simulink model "TST_RWSWV2"  (Simulink 10.1)
settings: Solver=FixedStepAuto  StartTime=0.0  StopTime=5.256e+6  FixedStep=1  RelTol=1e-3
libraries: LIB_ROT x3, vrlib x2, dspmathops x2, DYN x1
settings Model: Creator=WilTravis  LastModifiedBy=m_mam
settings DataIOCC: SaveFormat=Dataset
settings OptimizationCC: LifeSpan=auto
settings DebuggingCC: UnderspecifiedInitializationDetection=Simplified  MergeDetectMultiDrivingBlocksExec=error  SFUnexpectedBacktrackingDiag=error  SFNoUnconditionalDefaultTransitionDiag=error  SFExecutionAtInitializationDiag=warning
settings HardwareCC: ProdBitPerLong=64  ProdBitPerPointer=64  ProdBitPerSizeT=64  ProdBitPerPtrDiffT=64  ProdIntDivRoundTo=Zero  ProdEndianess=LittleEndian  ProdWordSize=64  ProdHWDeviceType=AMD->Athlon 64
settings ModelReferenceCC: PropagateSignalLabelsOutOfModel=on
settings CodeAppCC: StateflowObjectComments=off
settings GRTTargetCC: TargetLangStandard=C99 (ISO)  CombineOutputUpdateFcns=on  GRTInterface=off
settings ConfigComp: CovMetricSettings=dwe  CovHtmlReporting=off  CovSaveCumulativeToWorkspaceVar=off  CovSaveSingleToWorkspaceVar=off  CovExternalEMLEnable=on

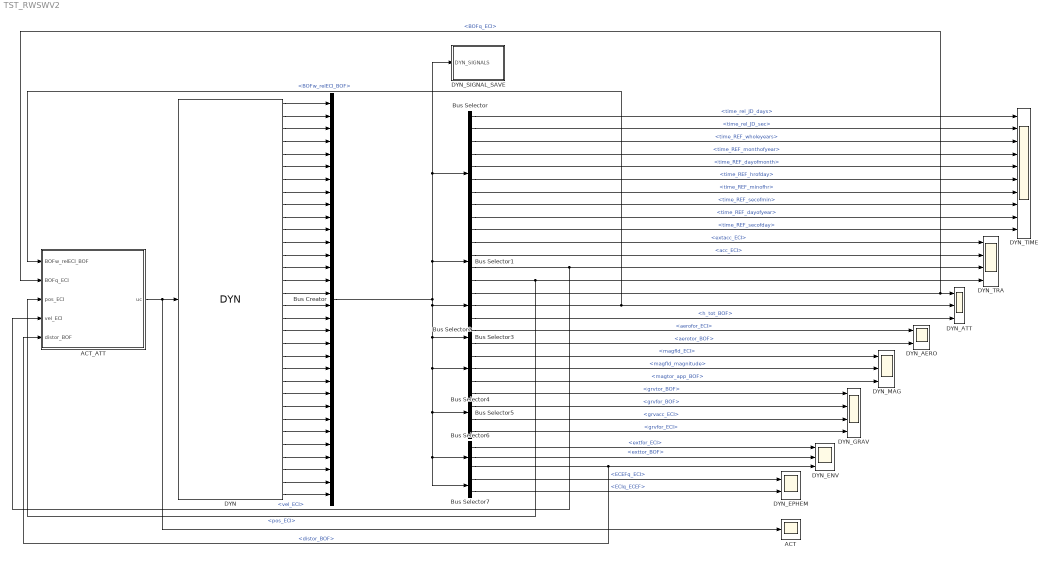
== system TST_RWSWV2 ==
  ACT : Scope
  ACT_ATT : Subsystem
  Bus Creator : BusCreator  Inputs=32
  Bus Selector : BusSelector  OutputSignals=time_rel_JD_days,time_rel_JD_sec,time_REF_wholeyears,time_REF_monthofyear,time_REF_dayofmonth,time_REF_hrofday,time_REF_minofhr,time_REF_secofmin,time_REF_dayofyear,time_REF_secofday
  Bus Selector1 : BusSelector  OutputSignals=extacc_ECI,acc_ECI,vel_ECI,pos_ECI
  Bus Selector2 : BusSelector  OutputSignals=BOFq_ECI,BOFw_relECI_BOF,h_tot_BOF
  Bus Selector3 : BusSelector  OutputSignals=aerofor_ECI,aerotor_BOF
  Bus Selector4 : BusSelector  OutputSignals=magfld_ECI,magfld_magnitude,magtor_app_BOF
  Bus Selector5 : BusSelector  OutputSignals=grvtor_BOF,grvfor_BOF,grvacc_ECI,grvfor_ECI
  Bus Selector6 : BusSelector  OutputSignals=extfor_ECI,exttor_BOF,distor_BOF
  Bus Selector7 : BusSelector  OutputSignals=ECEFq_ECI,ECIq_ECEF
  DYN : DYN/DYN  SystemSampleTime=-1  Latency=0  AutoFrameSizeCalculation=off
  DYN_AERO : Scope  NumInputPorts=2
  DYN_ATT : Scope  NumInputPorts=3
  DYN_ENV : Scope  NumInputPorts=3
  DYN_EPHEM : Scope  NumInputPorts=2
  DYN_GRAV : Scope  NumInputPorts=4
  DYN_MAG : Scope  NumInputPorts=3
  DYN_SIGNAL_SAVE : Subsystem
  DYN_TIME : Scope  NumInputPorts=10
  DYN_TRA : Scope  NumInputPorts=4
  wires:
  Bus Selector4/1 -> DYN_MAG/1  "<magfld_ECI>"
  Bus Selector1/2 -> DYN_TRA/2  "<acc_ECI>"
  Bus Selector/2 -> DYN_TIME/2  "<time_rel_JD_sec>"
  Bus Selector/6 -> DYN_TIME/6  "<time_REF_hrofday>"
  Bus Selector5/1 -> DYN_GRAV/1  "<grvtor_BOF>"
  Bus Selector1/3 -> ACT_ATT/4(vel_ECI), DYN_TRA/3  "<vel_ECI>"
  Bus Selector1/1 -> DYN_TRA/1  "<extacc_ECI>"
  Bus Selector2/1 -> ACT_ATT/2(BOFq_ECI), DYN_ATT/1  "<BOFq_ECI>"
  Bus Selector3/2 -> DYN_AERO/2  "<aerotor_BOF>"
  Bus Selector/3 -> DYN_TIME/3  "<time_REF_wholeyears>"
  Bus Selector5/2 -> DYN_GRAV/2  "<grvfor_BOF>"
  Bus Selector/4 -> DYN_TIME/4  "<time_REF_monthofyear>"
  Bus Selector5/3 -> DYN_GRAV/3  "<grvacc_ECI>"
  Bus Selector3/1 -> DYN_AERO/1  "<aerofor_ECI>"
  Bus Selector/1 -> DYN_TIME/1  "<time_rel_JD_days>"
  Bus Selector/10 -> DYN_TIME/10  "<time_REF_secofday>"
  Bus Selector/7 -> DYN_TIME/7  "<time_REF_minofhr>"
  Bus Selector/8 -> DYN_TIME/8  "<time_REF_secofmin>"
  Bus Selector2/3 -> DYN_ATT/3  "<h_tot_BOF>"
  Bus Selector1/4 -> ACT_ATT/3(pos_ECI), DYN_TRA/4  "<pos_ECI>"
  Bus Selector2/2 -> DYN_ATT/2, ACT_ATT/1(BOFw_relECI_BOF)  "<BOFw_relECI_BOF>"
  Bus Selector4/2 -> DYN_MAG/2  "<magfld_magnitude>"
  Bus Selector4/3 -> DYN_MAG/3  "<magtor_app_BOF>"
  Bus Selector/9 -> DYN_TIME/9  "<time_REF_dayofyear>"
  Bus Selector/5 -> DYN_TIME/5  "<time_REF_dayofmonth>"
  Bus Selector7/1 -> DYN_EPHEM/1  "<ECEFq_ECI>"
  Bus Selector7/2 -> DYN_EPHEM/2  "<ECIq_ECEF>"
  Bus Selector5/4 -> DYN_GRAV/4  "<grvfor_ECI>"
  Bus Selector6/1 -> DYN_ENV/1  "<extfor_ECI>"
  Bus Selector6/2 -> DYN_ENV/2  "<exttor_BOF>"
  DYN/1 -> Bus Creator/1
  DYN/2 -> Bus Creator/2
  DYN/3 -> Bus Creator/3
  DYN/4 -> Bus Creator/4
  DYN/5 -> Bus Creator/5
  DYN/6 -> Bus Creator/6
  DYN/7 -> Bus Creator/7
  DYN/8 -> Bus Creator/8
  DYN/9 -> Bus Creator/9
  DYN/10 -> Bus Creator/10
  DYN/11 -> Bus Creator/11
  DYN/12 -> Bus Creator/12
  DYN/13 -> Bus Creator/13
  DYN/14 -> Bus Creator/14
  DYN/15 -> Bus Creator/15
  DYN/16 -> Bus Creator/16
  DYN/17 -> Bus Creator/17
  DYN/18 -> Bus Creator/18
  DYN/19 -> Bus Creator/19
  DYN/20 -> Bus Creator/20
  DYN/21 -> Bus Creator/21
  DYN/22 -> Bus Creator/22
  DYN/23 -> Bus Creator/23
  DYN/24 -> Bus Creator/24
  DYN/25 -> Bus Creator/25
  DYN/26 -> Bus Creator/26
  DYN/27 -> Bus Creator/27
  DYN/28 -> Bus Creator/28
  DYN/29 -> Bus Creator/29
  DYN/30 -> Bus Creator/30
  Bus Creator/1 -> Bus Selector7/1, Bus Selector6/1, Bus Selector5/1, Bus Selector4/1, Bus Selector3/1, Bus Selector2/1, DYN_SIGNAL_SAVE/1(DYN_SIGNALS), Bus Selector/1, Bus Selector1/1
  DYN/31 -> Bus Creator/31
  ACT_ATT/1(uc) -> ACT/1, DYN/1
  DYN/32 -> Bus Creator/32
  Bus Selector6/3 -> ACT_ATT/5(distor_BOF), DYN_ENV/3  "<distor_BOF>"

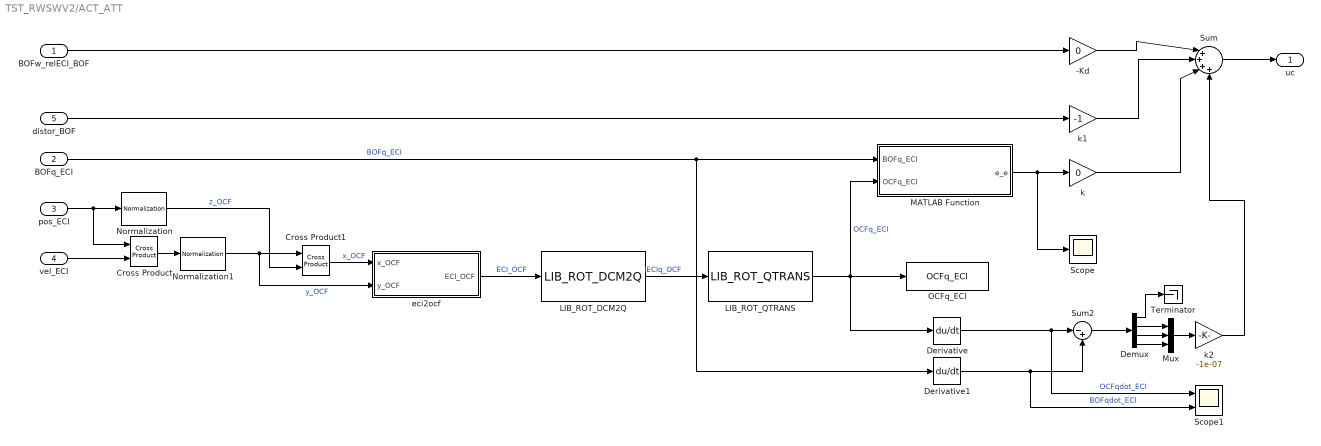
== system TST_RWSWV2/ACT_ATT ==
  BOFw_relECI_BOF : Inport
  BOFq_ECI : Inport  Port=2
  pos_ECI : Inport  Port=3
  vel_ECI : Inport  Port=4
  distor_BOF : Inport  Port=5
  -Kd : Gain  Gain=0
  Cross Product : vrlib/Utilities/Cross Product
  Cross Product1 : vrlib/Utilities/Cross Product
  Demux : Demux
  Derivative : Derivative
  Derivative1 : Derivative
  LIB_ROT_DCM2Q : LIB_ROT/LIB_ROT_DCM2Q
  LIB_ROT_QTRANS : LIB_ROT/LIB_ROT_QTRANS
  MATLAB Function : MATLAB Function  TreatAsAtomicUnit=on
  Mux : Mux  Inputs=3
  Normalization : dspmathops/Normalization  NormType=2-norm  Bias=1e-20  NormOver=Each column  Dimension=1  roundingMode=Floor  overflowMode=off  accumDataTypeStr=Inherit: Same as product output  accumLastDataTypeStr=Inherit: Same as product output  outputDataTypeStr=Inherit: Same as product output  outputMin=[]  outputMax=[]  outputLastDataTypeStr=Inherit: Same as product output
  Normalization1 : dspmathops/Normalization  NormType=2-norm  Bias=1e-20  NormOver=Each column  Dimension=1  roundingMode=Floor  overflowMode=off  accumDataTypeStr=Inherit: Same as product output  accumLastDataTypeStr=Inherit: Same as product output  outputDataTypeStr=Inherit: Same as product output  outputMin=[]  outputMax=[]  outputLastDataTypeStr=Inherit: Same as product output
  OCFq_ECI : ToWorkspace  VariableName=OCFq_ECI  SaveFormat=Structure With Time  SampleTime=-1
  Scope : Scope
  Scope1 : Scope  NumInputPorts=2
  Sum : Sum  Inputs=|++++
  Sum2 : Sum  Inputs=|-+
  Terminator : Terminator
  eci2ocf : MATLAB Function  TreatAsAtomicUnit=on
  k : Gain  Gain=0
  k1 : Gain  Gain=-1
  k2 : Gain  Gain=-1e-07
  uc : Outport
  wires:
  BOFw_relECI_BOF/1 -> -Kd/1
  BOFq_ECI/1 -> Derivative1/1, MATLAB Function/1(BOFq_ECI)  "BOFq_ECI"
  pos_ECI/1 -> Cross Product/1, Normalization/1
  vel_ECI/1 -> Cross Product/2
  Cross Product/1 -> Normalization1/1
  Normalization1/1 -> eci2ocf/2(y_OCF), Cross Product1/1  "y_OCF"
  Normalization/1 -> Cross Product1/2  "z_OCF"
  Cross Product1/1 -> eci2ocf/1(x_OCF)  "x_OCF"
  eci2ocf/1(ECI_OCF) -> LIB_ROT_DCM2Q/1  "ECI_OCF"
  LIB_ROT_DCM2Q/1 -> LIB_ROT_QTRANS/1  "ECIq_OCF"
  LIB_ROT_QTRANS/1 -> Derivative/1, OCFq_ECI/1, MATLAB Function/2(OCFq_ECI)  "OCFq_ECI"
  MATLAB Function/1(e_e) -> Scope/1, k/1
  -Kd/1 -> Sum/1
  Sum/1 -> uc/1
  k/1 -> Sum/3
  distor_BOF/1 -> k1/1
  k1/1 -> Sum/2
  Derivative/1 -> Scope1/1, Sum2/1  "OCFqdot_ECI"
  Derivative1/1 -> Scope1/2, Sum2/2  "BOFqdot_ECI"
  Demux/1 -> Terminator/1
  Sum2/1 -> Demux/1
  Demux/2 -> Mux/1
  Demux/3 -> Mux/2
  Demux/4 -> Mux/3
  Mux/1 -> k2/1
  k2/1 -> Sum/4

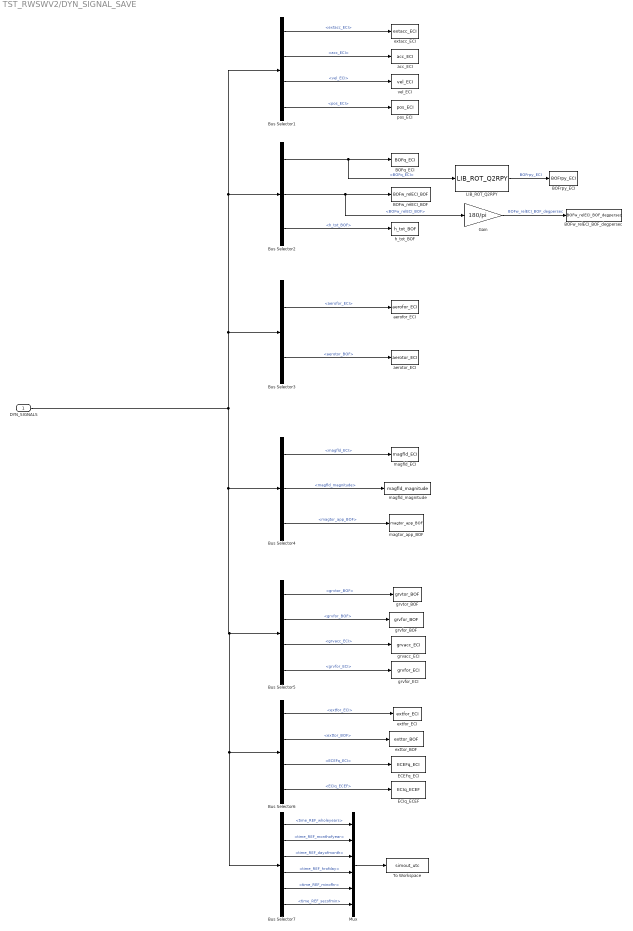
== system TST_RWSWV2/DYN_SIGNAL_SAVE ==
  DYN_SIGNALS : Inport
  BOFq_ECI : ToWorkspace  VariableName=BOFq_ECI  SaveFormat=Structure With Time  SampleTime=-1
  BOFrpy_ECI : ToWorkspace  VariableName=BOFrpy_ECI  SaveFormat=Structure With Time  SampleTime=-1
  BOFw_relECI_BOF : ToWorkspace  VariableName=BOFw_relECI_BOF  SaveFormat=Structure With Time  SampleTime=-1
  BOFw_relECI_BOF_degpersec : ToWorkspace  VariableName=BOFw_relECI_BOF_degpersec  SaveFormat=Structure With Time  SampleTime=-1
  Bus Selector1 : BusSelector  OutputSignals=extacc_ECI,acc_ECI,vel_ECI,pos_ECI
  Bus Selector2 : BusSelector  OutputSignals=BOFq_ECI,BOFw_relECI_BOF,h_tot_BOF
  Bus Selector3 : BusSelector  OutputSignals=aerofor_ECI,aerotor_BOF
  Bus Selector4 : BusSelector  OutputSignals=magfld_ECI,magfld_magnitude,magtor_app_BOF
  Bus Selector5 : BusSelector  OutputSignals=grvtor_BOF,grvfor_BOF,grvacc_ECI,grvfor_ECI
  Bus Selector6 : BusSelector  OutputSignals=extfor_ECI,exttor_BOF,ECEFq_ECI,ECIq_ECEF
  Bus Selector7 : BusSelector  OutputSignals=time_REF_wholeyears,time_REF_monthofyear,time_REF_dayofmonth,time_REF_hrofday,time_REF_minofhr,time_REF_secofmin
  ECEFq_ECI : ToWorkspace  VariableName=ECEFq_ECI  SaveFormat=Structure With Time  SampleTime=-1
  ECIq_ECEF : ToWorkspace  VariableName=ECIq_ECEF  SaveFormat=Structure With Time  SampleTime=-1
  Gain : Gain  Gain=180/pi
  LIB_ROT_Q2RPY : LIB_ROT/LIB_ROT_Q2RPY
  Mux : Mux  Inputs=6
  To Workspace : ToWorkspace  VariableName=simout_utc  SaveFormat=Timeseries  SampleTime=-1
  acc_ECI : ToWorkspace  VariableName=acc_ECI  SaveFormat=Structure With Time  SampleTime=-1
  aerofor_ECI : ToWorkspace  VariableName=aerofor_ECI  SaveFormat=Structure With Time  SampleTime=-1
  aerotor_ECI : ToWorkspace  VariableName=aerotor_ECI  SaveFormat=Structure With Time  SampleTime=-1
  extacc_ECI : ToWorkspace  VariableName=extacc_ECI  SaveFormat=Structure With Time  SampleTime=-1
  extfor_ECI : ToWorkspace  VariableName=extfor_ECI  SaveFormat=Structure With Time  SampleTime=-1
  exttor_BOF : ToWorkspace  VariableName=exttor_BOF  SaveFormat=Structure With Time  SampleTime=-1
  grvacc_ECI : ToWorkspace  VariableName=grvacc_ECI  SaveFormat=Structure With Time  SampleTime=-1
  grvfor_BOF : ToWorkspace  VariableName=grvfor_BOF  SaveFormat=Structure With Time  SampleTime=-1
  grvfor_ECI : ToWorkspace  VariableName=grvfor_ECI  SaveFormat=Structure With Time  SampleTime=-1
  grvtor_BOF : ToWorkspace  VariableName=grvtor_BOF  SaveFormat=Structure With Time  SampleTime=-1
  h_tot_BOF : ToWorkspace  VariableName=h_tot_BOF  SaveFormat=Structure With Time  SampleTime=-1
  magfld_ECI : ToWorkspace  VariableName=magfld_ECI  SaveFormat=Structure With Time  SampleTime=-1
  magfld_magnitude : ToWorkspace  VariableName=magfld_magnitude  SaveFormat=Structure With Time  SampleTime=-1
  magtor_app_BOF : ToWorkspace  VariableName=magtor_app_BOF  SaveFormat=Structure With Time  SampleTime=-1
  pos_ECI : ToWorkspace  VariableName=pos_ECI  SaveFormat=Structure With Time  SampleTime=-1
  vel_ECI : ToWorkspace  VariableName=vel_ECI  SaveFormat=Structure With Time  SampleTime=-1
  wires:
  DYN_SIGNALS/1 -> Bus Selector7/1, Bus Selector6/1, Bus Selector5/1, Bus Selector4/1, Bus Selector1/1, Bus Selector2/1, Bus Selector3/1
  Bus Selector1/1 -> extacc_ECI/1  "<extacc_ECI>"
  Bus Selector1/2 -> acc_ECI/1  "<acc_ECI>"
  Bus Selector1/3 -> vel_ECI/1  "<vel_ECI>"
  Bus Selector1/4 -> pos_ECI/1  "<pos_ECI>"
  Bus Selector2/1 -> LIB_ROT_Q2RPY/1, BOFq_ECI/1  "<BOFq_ECI>"
  Bus Selector2/2 -> Gain/1, BOFw_relECI_BOF/1  "<BOFw_relECI_BOF>"
  Bus Selector2/3 -> h_tot_BOF/1  "<h_tot_BOF>"
  Bus Selector3/1 -> aerofor_ECI/1  "<aerofor_ECI>"
  Bus Selector3/2 -> aerotor_ECI/1  "<aerotor_BOF>"
  Bus Selector4/1 -> magfld_ECI/1  "<magfld_ECI>"
  Bus Selector4/2 -> magfld_magnitude/1  "<magfld_magnitude>"
  Bus Selector4/3 -> magtor_app_BOF/1  "<magtor_app_BOF>"
  Bus Selector5/4 -> grvfor_ECI/1  "<grvfor_ECI>"
  Bus Selector5/3 -> grvacc_ECI/1  "<grvacc_ECI>"
  Bus Selector5/2 -> grvfor_BOF/1  "<grvfor_BOF>"
  Bus Selector5/1 -> grvtor_BOF/1  "<grvtor_BOF>"
  Bus Selector6/3 -> ECEFq_ECI/1  "<ECEFq_ECI>"
  Bus Selector6/4 -> ECIq_ECEF/1  "<ECIq_ECEF>"
  Bus Selector6/1 -> extfor_ECI/1  "<extfor_ECI>"
  Bus Selector6/2 -> exttor_BOF/1  "<exttor_BOF>"
  LIB_ROT_Q2RPY/1 -> BOFrpy_ECI/1  "BOFrpy_ECI"
  Gain/1 -> BOFw_relECI_BOF_degpersec/1  "BOFw_relECI_BOF_degpersec"
  Bus Selector7/1 -> Mux/1  "<time_REF_wholeyears>"
  Bus Selector7/2 -> Mux/2  "<time_REF_monthofyear>"
  Bus Selector7/3 -> Mux/3  "<time_REF_dayofmonth>"
  Bus Selector7/4 -> Mux/4  "<time_REF_hrofday>"
  Bus Selector7/5 -> Mux/5  "<time_REF_minofhr>"
  Bus Selector7/6 -> Mux/6  "<time_REF_secofmin>"
  Mux/1 -> To Workspace/1

== matlab function ACT_ATT/MATLAB Function ==
  data: BOFq_ECI input double; OCFq_ECI input double; e_e output double
function e_e = qerror(BOFq_ECI,OCFq_ECI)

n_d = OCFq_ECI(1);
e_d = [OCFq_ECI(2);OCFq_ECI(3);OCFq_ECI(4)];

q_error = [-e_d n_d*eye(3)-VecCross(e_d);
    n_d e_d']*BOFq_ECI;

e_e = [q_error(2);q_error(3);q_error(4)];

== matlab function ACT_ATT/eci2ocf ==
  data: x_OCF input double; ECI_OCF output double; y_OCF input double
function ECI_OCF = eci2ocf(x_OCF, y_OCF)

ECI_OCF = [x_OCF';y_OCF';y_OCF'];
